simulink model "SystemInterconnectionsSimulator"  (R2023b)
settings: Solver=VariableStepAuto  StartTime=0.0  StopTime=10  MaxStep=0.001  MinStep=0.00001  RelTol=1e-6
settings Model: Creator=Tefo  LastModifiedBy=Tefo

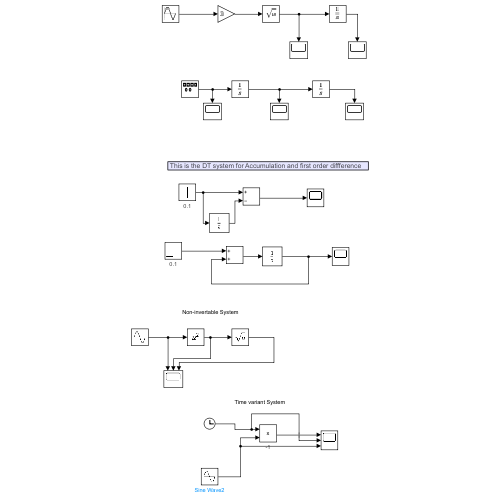
[thumbnail: Simulink's stored preview of the top-level diagram]
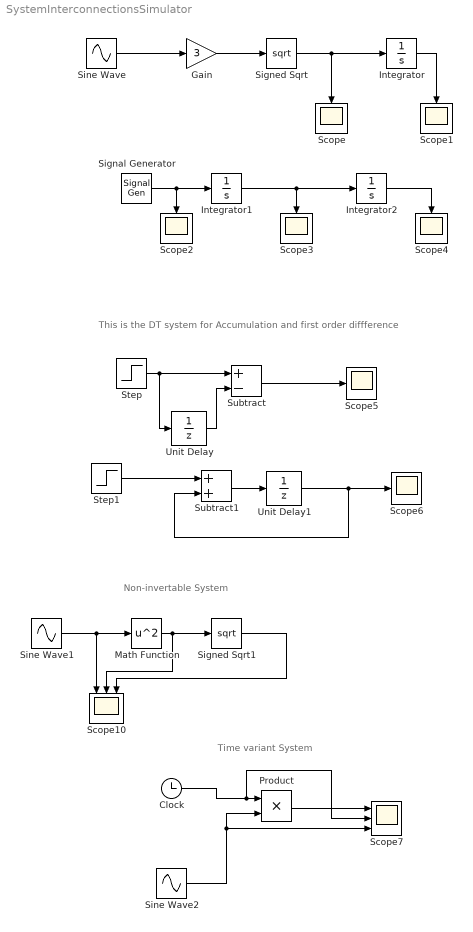
== system SystemInterconnectionsSimulator ==
  note: Non-invertable System
  note: This is the DT system for Accumulation and first order diffference
  note: Time variant System
  Clock : Clock
  Gain : Gain  Gain=3
  Integrator : Integrator
  Integrator1 : Integrator
  Integrator2 : Integrator
  Math Function : Math  Operator=square
  Product : Product
      settings: AttributesFormatString=%<SampleTime>
  Scope{,1..6} (7 alike) : Scope
  Scope10 : Scope  NumInputPorts=3
  Scope7 : Scope  NumInputPorts=3
  Signal Generator : SignalGenerator  WaveForm=random  Units=rad/sec
  Signed Sqrt : Sqrt
  Signed Sqrt1 : Sqrt
  Sine Wave : Sin  SampleTime=0
  Sine Wave1 : Sin  Frequency=5  SampleTime=0
  Sine Wave2 : Sin  Amplitude=3  Frequency=5  SampleTime=0
  Step : Step  SampleTime=0.1
      settings: AttributesFormatString=%<SampleTime>
  Step1 : Step  SampleTime=0.1
      settings: AttributesFormatString=%<SampleTime>
  Subtract : Sum  Inputs=+-
  Subtract1 : Sum
  Unit Delay : UnitDelay  SampleTime=-1  HasFrameUpgradeWarning=on
  Unit Delay1 : UnitDelay  SampleTime=-1  HasFrameUpgradeWarning=on
  wires:
  Sine Wave/1 -> Gain/1
  Gain/1 -> Signed Sqrt/1
  Signed Sqrt/1 -> Integrator/1, Scope/1
  Integrator/1 -> Scope1/1
  Signal Generator/1 -> Integrator1/1, Scope2/1
  Integrator1/1 -> Integrator2/1, Scope3/1
  Integrator2/1 -> Scope4/1
  Step/1 -> Unit Delay/1, Subtract/1
  Unit Delay/1 -> Subtract/2
  Subtract/1 -> Scope5/1
  Step1/1 -> Subtract1/1
  Subtract1/1 -> Unit Delay1/1
  Unit Delay1/1 -> Scope6/1, Subtract1/2
  Math Function/1 -> Scope10/2, Signed Sqrt1/1
  Signed Sqrt1/1 -> Scope10/3
  Sine Wave1/1 -> Math Function/1, Scope10/1
  Clock/1 -> Scope7/2, Product/1
  Sine Wave2/1 -> Scope7/3, Product/2
  Product/1 -> Scope7/1
